simulink model "MAVROS_Move"  (R2023a)
settings: Solver=FixedStepAuto  StartTime=0.0  StopTime=Inf  RelTol=1e-3
model workspace (MAT data in the model file):
  SL_ROS_VariableLengthArrays_MaxSizes.CommonInfo.ArrayTruncateAction = 'EmitWarning'
  SL_ROS_VariableLengthArrays_MaxSizes.MsgTypeMap = containers.Map
  SL_ROS_VariableLengthArrays_MaxSizes.MsgTypeMap.serialization.keys = {'sensor_msgs/LaserScan'}
  SL_ROS_VariableLengthArrays_MaxSizes.MsgTypeMap.serialization.values{1}(1).PropertyName = 'Intensities'
  SL_ROS_VariableLengthArrays_MaxSizes.MsgTypeMap.serialization.values{1}(1).DataType = 'single'
  SL_ROS_VariableLengthArrays_MaxSizes.MsgTypeMap.serialization.values{1}(1).MaxLength = 360
  SL_ROS_VariableLengthArrays_MaxSizes.MsgTypeMap.serialization.values{1}(2).PropertyName = 'Ranges'
  SL_ROS_VariableLengthArrays_MaxSizes.MsgTypeMap.serialization.values{1}(2).DataType = 'single'
  SL_ROS_VariableLengthArrays_MaxSizes.MsgTypeMap.serialization.values{1}(2).MaxLength = 360
  SL_ROS_VariableLengthArrays_MaxSizes.MsgTypeMap.serialization.uniformity = 0
  SL_ROS_VariableLengthArrays_MaxSizes.MsgTypeMap.serialization.keyType = 'char'
  SL_ROS_VariableLengthArrays_MaxSizes.MsgTypeMap.serialization.valueType = 'any'
undefined symbols (not defined in the file or in its folder): Twist
libraries: robotlib x7, aerolibanimutils x1
settings Model: Creator=cesf9  LastModifiedBy=cesf9
settings OptimizationCC: EnhancedBackFolding=on  PassReuseOutputArgsAs=Individual arguments  ZeroExternalMemoryAtStartup=off  ZeroInternalMemoryAtStartup=off  MaxStackSize=64  OptimizeBlockOrder=speed  DifferentSizesBufferReuse=on  OptimizationCustomize=off  EfficientTunableParamExpr=on
settings DebuggingCC: ParameterTunabilityLossMsg=error
settings HardwareCC: ProdBitPerPointer=32  ProdBitPerSizeT=32  ProdBitPerPtrDiffT=32  ProdLargestAtomicFloat=None  ProdIntDivRoundTo=Undefined  ProdEndianess=Unspecified  ProdWordSize=32  ProdHWDeviceType=Generic->Unspecified (assume 32-bit Generic)
settings SFSimCC: MATLABDynamicMemAlloc=off
settings RTWCC: Description=Embedded Coder  SystemTargetFile=ert.tlc  HardwareBoard=Robot Operating System (ROS)  TLCOptions="-aInlineSetEventsForThisBaseRateFcn=TLC_FALSE -aSuppressMultiTaskScheduler=TLC_FALSE  -aRateBasedStepFcn=0"  TemplateMakefile=ert_default_tmf  Toolchain=Catkin  TargetLang=C++
settings CodeAppCC: ForceParamTrailComments=on  IgnoreCustomStorageClasses=off  OperatorAnnotations=on  SimulinkDataObjDesc=on  SFDataObjDesc=on  InsertBlockDesc=on

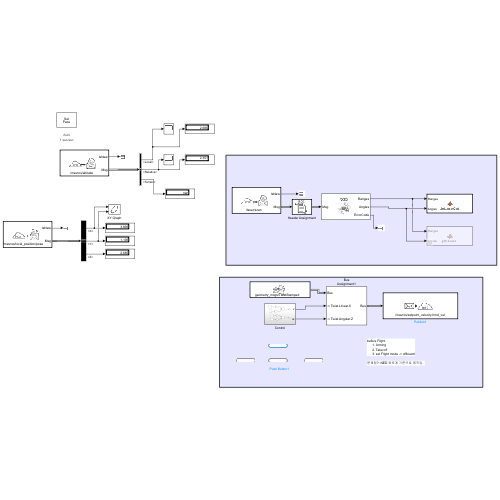
[thumbnail: Simulink's stored preview of the top-level diagram]
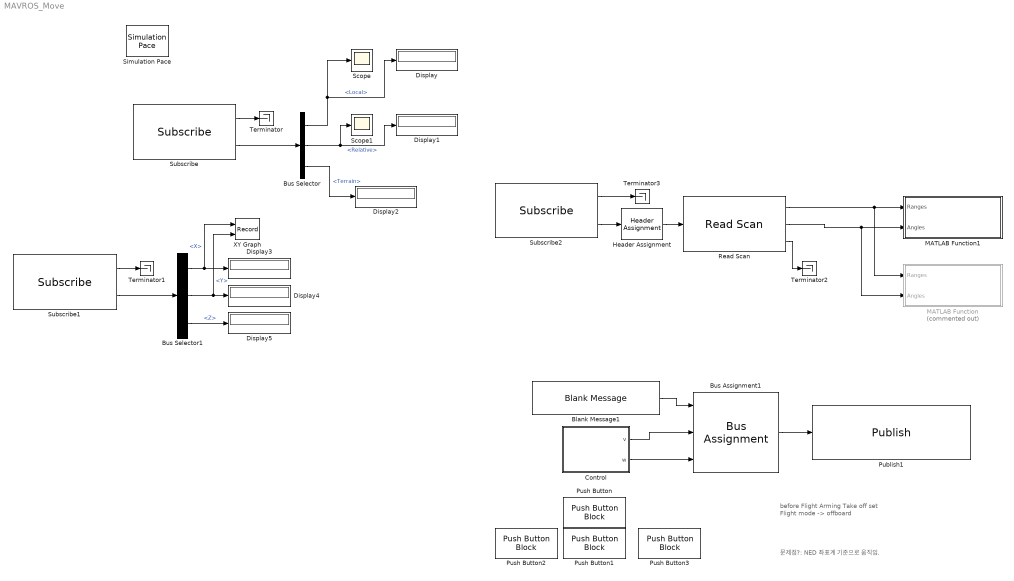
== system MAVROS_Move ==
  note: 문제점?: NED 좌표계 기준으로 움직임.
  note: before Flight
      | Arming
      | Take off
      | set Flight mode -> offboard
  Blank Message1 : robotlib/Blank Message  messageClass=Message  entityType=geometry_msgs/TwistStamped  messageType=geometry_msgs/TwistStamped  SampleTime=0.1  legacyBusStruct=off
  Bus Assignment1 : BusAssignment  AssignedSignals=Twist.Linear.X,Twist.Angular.Z
  Bus Selector : BusSelector  OutputSignals=Local,Relative,Terrain
  Bus Selector1 : BusSelector  OutputSignals=Pose.Position.X,Pose.Position.Y,Pose.Position.Z
  Control : Subsystem
  Display{,1..5} (6 alike) : Display
  Header Assignment : robotlib/Header Assignment  SetFrameID=on  FrameID=rplidar_link  InsertTimeStamp=off  SetHeaderFieldName=Use the default Header field name  HeaderFieldName=Header
  MATLAB Function : MATLAB Function  Commented=on  TreatAsAtomicUnit=on
  MATLAB Function1 : MATLAB Function  TreatAsAtomicUnit=on
  Publish1 : robotlib/Publish  topicSource=Select from ROS network  topic=/mavros/setpoint_velocity/cmd_vel  messageType=geometry_msgs/TwistStamped  legacyBusStruct=off  messageQueueLength=1
  Push Button : PushButtonBlock  ButtonText=Fwd  OffValue=0.000000
  Push Button1 : PushButtonBlock  ButtonText=Back  OffValue=0.000000
  Push Button2 : PushButtonBlock  ButtonText=Left  OffValue=0.000000
  Push Button3 : PushButtonBlock  ButtonText=Right  OffValue=0.000000
  Read Scan : robotlib/Read Scan  MaximumArrayLength=360  ShowAnglesOutput=on  ShowIntensityOutput=off  ShowErrorCodeOutput=on  VariableSizeOutputs=off
  Scope : Scope
  Scope1 : Scope
  Simulation Pace : aerolibanimutils/Simulation Pace  SimulationPace=1  SleepMode=Auto  OutputPaceError=off  SampleTime=1/30
  Subscribe : robotlib/Subscribe  topicSource=Select from ROS network  topic=/mavros/altitude  messageType=mavros_msgs/Altitude  SampleTime=-1  legacyBusStruct=off  messageQueueLength=1
  Subscribe1 : robotlib/Subscribe  topicSource=Select from ROS network  topic=/mavros/local_position/pose  messageType=geometry_msgs/PoseStamped  SampleTime=-1  legacyBusStruct=off  messageQueueLength=1
  Subscribe2 : robotlib/Subscribe  topicSource=Select from ROS network  topic=/laser/scan  messageType=sensor_msgs/LaserScan  SampleTime=-1  legacyBusStruct=off  messageQueueLength=1
  Terminator{,1..3} (4 alike) : Terminator
  XY Graph : Record  FileSettingsInternal="{\"entries\":[{\"content\":{\"excelSettings\":{\"content\":{},\"type\":\"Streamout.ExcelSettings\"}},\"type\":\"Streamout.FileSettingStorage\",\"uuid\":\"\"}],\"packageUris\":[\"http:\\/\\/schema.mathworks.com\\/mf0\\/streamout_blocks\\/R2020a\"],\"version\":\"1.0\"}"  Layout=[1 1]  SignalsInternal="{\"entries\":[{\"content\":{\"signals\":[{\"content\":{\"blockPath\":[],\"dimensions\":[1],\"domain\":\"\",\"lineColor\":\"#a2142f\",\"plots\":[1],\"port\":1,\"signalID\":338,\"signalName\":\"XY Graph:1\"},\"type\":\"RecordBlkView.Signal\",\"uuid\":\"\"},{\"content\":{\"blockPath\":[],\"dimensions\":[1],\"domain\":\"\",\"lineColor\":\"#139fff\",\"plots\":[1],\"port\":2,\"signalID\":341,\"signalName\":\"XY Graph:2\"},\"type\":\"RecordBlkView.Signal\",\"uuid\":\"\"}]},\"type\":\"RecordBlkView.InputSignals\",\"uuid\":\"\"}],\"packageUris\":[\"http:\\/\\/schema.mathworks.com\\/mf0\\/streamout_blocks\\/R2020a\"],\"version\":\"1.0\"}"  VisualizationBindings="{\"xyplotplugin\":{\"info\":[{\"series\":[{\"bindingParametersList\":[{\"parameter\":\"X-Axis\",\"signalID\":338,\"signalName\":\"XY Graph:1\"},{\"parameter\":\"Y-Axis\",\"signalID\":341,\"signalName\":\"XY Graph:2\"}],\"seriesID\":58420}],\"subplotID\":1}]}}"  CompatibilityTag=XY
  wires:
  Subscribe/2 -> Bus Selector/1
  Bus Selector/1 -> Scope/1, Display/1  "<Local>"
  Bus Selector/2 -> Scope1/1, Display1/1  "<Relative>"
  Bus Selector/3 -> Display2/1  "<Terrain>"
  Subscribe/1 -> Terminator/1
  Subscribe1/1 -> Terminator1/1
  Subscribe1/2 -> Bus Selector1/1
  Bus Selector1/1 -> XY Graph/1, Display3/1  "<X>"
  Bus Selector1/2 -> XY Graph/2, Display4/1  "<Y>"
  Bus Selector1/3 -> Display5/1  "<Z>"
  Read Scan/1 -> MATLAB Function/1(Ranges), MATLAB Function1/1(Ranges)
  Read Scan/2 -> MATLAB Function/2(Angles), MATLAB Function1/2(Angles)
  Subscribe2/2 -> Header Assignment/1
  Header Assignment/1 -> Read Scan/1
  Read Scan/3 -> Terminator2/1
  Subscribe2/1 -> Terminator3/1
  Bus Assignment1/1 -> Publish1/1
  Control/2(w) -> Bus Assignment1/3
  Control/1(v) -> Bus Assignment1/2
  Blank Message1/1 -> Bus Assignment1/1

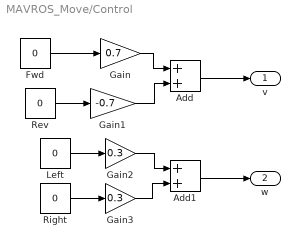
== system MAVROS_Move/Control ==
  Add : Sum
  Add1 : Sum
  Fwd : Constant  Value=0
  Gain : Gain  Gain=0.7
  Gain1 : Gain  Gain=-0.7
  Gain2 : Gain  Gain=0.3
  Gain3 : Gain  Gain=0.3
  Left : Constant  Value=0
  Rev : Constant  Value=0
  Right : Constant  Value=0
  v : Outport
  w : Outport  Port=2
  wires:
  Rev/1 -> Gain1/1
  Add/1 -> v/1
  Left/1 -> Gain2/1
  Fwd/1 -> Gain/1
  Right/1 -> Gain3/1
  Add1/1 -> w/1
  Gain/1 -> Add/1
  Gain1/1 -> Add/2
  Gain2/1 -> Add1/1
  Gain3/1 -> Add1/2

== matlab function MAVROS_Move/MATLAB Function ==
  data: Ranges input; Angles input
function plotLaser(Ranges, Angles)
coder.extrinsic('polarplot');
persistent p;
if isempty(p)
    p = polarplot(0, 0, '.');
    set(gca, 'ThetaZeroLocation', 'top', 'ThetaLim', [-135 135], ...
        'RAxisLocation', 0, 'RLim', [0 10]);
end
if ishandle(p)
    set(p, 'ThetaData', Angles);
    set(p, 'RData', Ranges);
    drawnow limitrate;
end

== matlab function MAVROS_Move/MATLAB Function1 ==
  data: Ranges input; Angles input
function plotLaserCart(Ranges, Angles)
coder.extrinsic('plot');
persistent p;

X = Ranges .* sin(Angles);
Y = Ranges .* -cos(Angles);

if isempty(p)
    p = plot(0, 0, '.');
    set(gca,'XLim',[-5 5],'YLim',[-5 5])
end
if ishandle(p)
    set(p, 'XData', X);
    set(p, 'YData', Y);
    drawnow limitrate;
end
